simulink model "ExampleDemo2"  (Simulink 5.0)
settings: Solver=ode45  StartTime=0.0  StopTime=1.0  RelTol=1e-3
values from neighbouring files (symbols this model uses):
  den = [1]    [dab1.m]    (also in dab1o.m)
  dx = 0    [dab1.m]    (also in dab1o.m)
  num = [1]    [dab1.m]    (also in dab1o.m)
settings Model: LastModifiedBy=Praveen

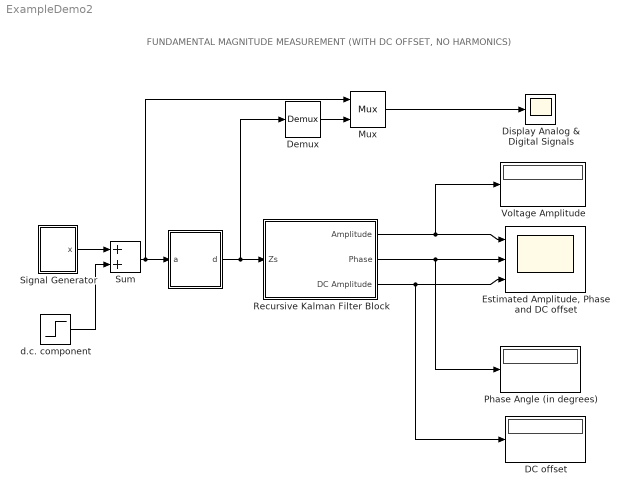
== system ExampleDemo2 ==
  note: FUNDAMENTAL MAGNITUDE MEASUREMENT (WITH DC OFFSET, NO HARMONICS)
  "  " : Subsystem  mask(Data Adquisition Board){filter=on, approx=Butterworth, order=3, numerator=[], denominator=[], freq=180, resdis=on, vertres=8, xmax=100, winsize=1, G=1.0, fs=60*20}
      mask prompts: filter "Disable Analog Filter"; approx "Filter approximation"; numerator "Free expression filter: numerator(descending order of s)"; denominator "Free expression filter: denominator:"; freq "Cut-off frequency"; resdis "Disable Vertical Resolution"; vertres "Vertical Resolution: No. of bits"; xmax "Vertical Resolution: signal range"; winsize "Window size"; G "Gain"; fs "Sampling frequency"
      mask help: Takes the instantaneous value of the input signal and convert it to the data window of samples.
      mask init:
      | dab1
      mask Help: web(['file:///' which('dab.html')]);
      mask StyleString: checkbox,popup(Bessel|Tschebyscheff|Butterworth|free expression),popup(2|3|4),edit,edit,edit,checkbox,popup(8|12|16),edit,edit,edit,edit
      mask Display: disp('DAB')
  DC offset : Display
  Demux : Demux  Outputs=1
  Display Analog & Digital Signals : Scope
      settings: TickLabels=on  TimeRange=1  YMin=-1.6  YMax=1.6  DataFormat=Array
  "Estimated Amplitude, Phase and DC offset" : Scope  NumInputPorts=3
      settings: TickLabels=on  TimeRange=1  YMin=0~-200~-0.2  YMax=1.4~200~0.6000000000000001
  Mux : Mux  Inputs=2
  Phase Angle (in degrees) : Display
  Recursive Kalman Filter Block : Subsystem  mask(Kalman Block){f=60, Fs=32, X0=[0;0;0], C=[1 0 1], sigman=0.01, sigmav=0.005, M=[(0.24^2) 0 0;0 (0.24^2) 0;0 0 (0.24^2)], lambda=0.001}
      mask prompts: f "Fundamental Frequency of Input Signal (f) in Hz"; Fs "Sampling Frequency (Fs) in samples per second"; X0 "Initial State (x0)"; C "Voltage-Phasor relation matrix (C)"; sigman "Measurement Noise Variance (Sigma n)"; sigmav "Process noise variance (Sigma v)"; M "Single step transition error covariance (M)"; lambda "Decaying DC Parameter (lambda)"
      mask help:
      | Measures the Phasor voltage values using the Kalman filter.
      | The input to the block is 'Zs(n)', the signal at time nT. 'f' is the fundamental frequency of the signal, and the harmonics are assumed to be integral multiple of this.
      | 'C' is the ralationship between voltage and phasor values. The default value is [1,0,1] assuming zero imaginary component and non-zero DC component.
      | Measurement noise variance 'sigman' models the noise during the voltage measurement.
      | Process variance 'sigmav' denotes the variation in the measurement of voltage values.
      | 'M' denotes the single step variation
      | Decaying DC component models the decreasing nature of the DC.
  Signal Generator : Subsystem  mask(Signal Generator){A1=1, f1=60, A2=0, f2=2*60, A3=0, f3=5*60, tstart=1.5/60}
      mask prompts: A1 "Amplitude 1"; f1 "Frequency 1 [Hz]"; A2 "Amplitude 2"; f2 "Frequency 2 [Hz]"; A3 "Amplitude 3"; f3 "Frequency 3 [Hz]"; tstart "Start time [sec]"
  Sum : Sum  SaturateOnIntegerOverflow=on  InputSameDT=on
  Voltage Amplitude : Display
  d.c. component : Step  Time=1.5/60  After=0.5
  wires:
  Sum/1 -> "  "/1(a), Mux/1
  d.c. component/1 -> Sum/2
  Signal Generator/1(x) -> Sum/1
  Mux/1 -> Display Analog & Digital Signals/1
  Demux/1 -> Mux/2
  "  "/1(d) -> Demux/1, Recursive Kalman Filter Block/1(Zs)
  Recursive Kalman Filter Block/2(Phase) -> "Estimated Amplitude, Phase and DC offset"/2, Phase Angle (in degrees)/1
  Recursive Kalman Filter Block/1(Amplitude) -> Voltage Amplitude/1, "Estimated Amplitude, Phase and DC offset"/1
  Recursive Kalman Filter Block/3(DC Amplitude) -> DC offset/1, "Estimated Amplitude, Phase and DC offset"/3

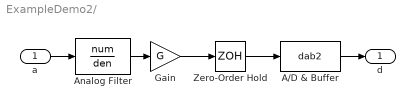
== system ExampleDemo2/   ==
  a : Inport
  A/D & Buffer : S-Function  FunctionName=dab2  Parameters=winsize,fs,dx,resdis
  Analog Filter : TransferFcn  Numerator=num  Denominator=den
  Gain : Gain  Gain=G  SaturateOnIntegerOverflow=on
  Zero-Order Hold : ZeroOrderHold  SampleTime=1/fs
  d : Outport  InitialOutput=[zeros(winsize,1)]
  wires:
  Analog Filter/1 -> Gain/1
  Gain/1 -> Zero-Order Hold/1
  Zero-Order Hold/1 -> A/D & Buffer/1
  a/1 -> Analog Filter/1
  A/D & Buffer/1 -> d/1

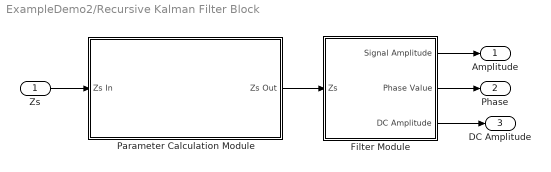
== system ExampleDemo2/Recursive Kalman Filter Block ==
  Zs : Inport
  Filter Module : Subsystem  Priority=2
  Parameter Calculation Module : Subsystem  Priority=1
      mask Display:
      | disp('PARAMETER MODULE');
      | port_label('input',1,'Zs in');
      | port_label('output',1,'Zs out');
  Amplitude : Outport
  Phase : Outport  Port=2
  DC Amplitude : Outport  Port=3
  wires:
  Zs/1 -> Parameter Calculation Module/1(Zs In)
  Parameter Calculation Module/1(Zs Out) -> Filter Module/1(Zs)
  Filter Module/1(Signal Amplitude) -> Amplitude/1
  Filter Module/3(DC Amplitude) -> DC Amplitude/1
  Filter Module/2(Phase Value) -> Phase/1

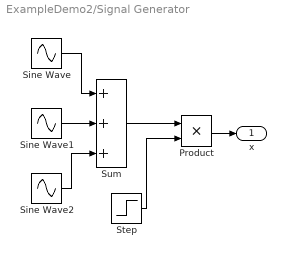
== system ExampleDemo2/Signal Generator ==
  Product : Product  SaturateOnIntegerOverflow=on  InputSameDT=on
  Sine Wave : Sin  Amplitude=A1  Frequency=f1*2*pi  SampleTime=0
  Sine Wave1 : Sin  Amplitude=A2  Frequency=f2*2*pi  SampleTime=0
  Sine Wave2 : Sin  Amplitude=A3  Frequency=f3*2*pi  SampleTime=0
  Step : Step  Time=tstart
  Sum : Sum  Inputs=+++  SaturateOnIntegerOverflow=on  InputSameDT=on
  x : Outport  InitialOutput=0
  wires:
  Sine Wave/1 -> Sum/1
  Sine Wave1/1 -> Sum/2
  Sine Wave2/1 -> Sum/3
  Sum/1 -> Product/1
  Step/1 -> Product/2
  Product/1 -> x/1

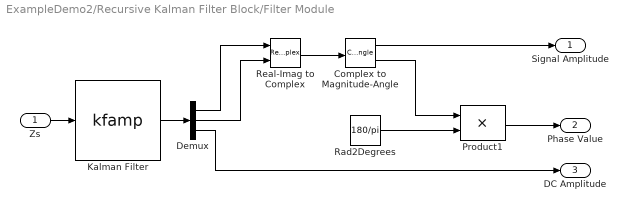
== system ExampleDemo2/Recursive Kalman Filter Block/Filter Module ==
  Zs : Inport
  Complex to Magnitude-Angle : ComplexToMagnitudeAngle
  Demux : Demux  Outputs=3
  Kalman Filter : S-Function  Priority=2  FunctionName=kfamp  Parameters=X0 C M
      mask Type: Kalman Filter Block
  Product1 : Product  ShowAdditionalParam=on  SaturateOnIntegerOverflow=on
  Rad2Degrees : Constant  Value=180/pi
  Real-Imag to Complex : RealImagToComplex
  Signal Amplitude : Outport
  Phase Value : Outport  Port=2
  DC Amplitude : Outport  Port=3
  wires:
  Zs/1 -> Kalman Filter/1
  Kalman Filter/1 -> Demux/1
  Demux/1 -> Real-Imag to Complex/1
  Demux/2 -> Real-Imag to Complex/2
  Demux/3 -> DC Amplitude/1
  Product1/1 -> Phase Value/1
  Real-Imag to Complex/1 -> Complex to Magnitude-Angle/1
  Complex to Magnitude-Angle/1 -> Signal Amplitude/1
  Rad2Degrees/1 -> Product1/2
  Complex to Magnitude-Angle/2 -> Product1/1

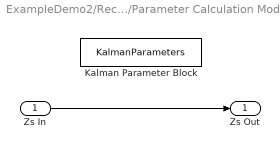
== system ExampleDemo2/Recursive Kalman Filter Block/Parameter Calculation Module ==
  Zs In : Inport
  Kalman Parameter Block : S-Function  Priority=1  FunctionName=KalmanParameters  Parameters=Fs f sigman sigmav M lambda
  Zs Out : Outport
  wires:
  Zs In/1 -> Zs Out/1
